simulink subsystem "EP_EmpennageForceMoment"  (R2025a)
settings: Solver=VariableStepAuto  StartTime=0.0  StopTime=10.0  RelTol=1e-3
undefined symbols (not defined in the file): EP_AirDensity_P, EP_CoGPos_P, EP_FinArea_P, EP_FinHeight_P, EP_FinLiftCoeffLim_P, EP_FinLiftSlope_P, EP_FinPos_P, EP_FinSetAng_P, EP_OutOfWakeAzimuth_P, EP_RotorRadius_P, EP_SkewAngleLwrLim_P, EP_SkewAngleUpprLim_P, EP_TailPlaneArea_P, EP_TailPlaneAzimuth_P, EP_TailPlaneLiftCoeffLim_P, EP_TailPlaneLiftSlope_P, EP_TailPlanePos_P, EP_TailPlaneSetAng_P, EP_WakeInitialInfluence_P
settings Model: DataDictionary=Empennage.sldd  EnableAccessToBaseWorkspace=off  DefaultTestHarness=EP_EmpennageForceMoment_Harness1  Creator=Admin  LastModifiedBy=Admin

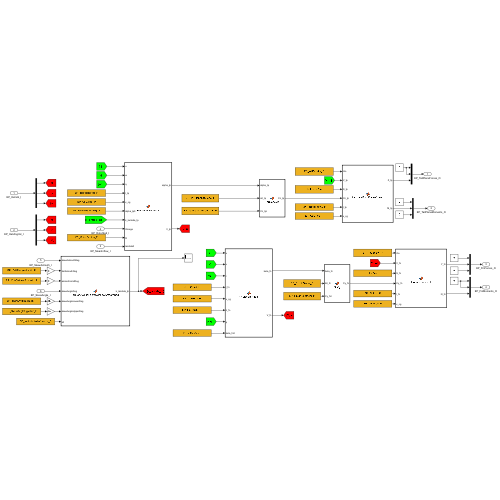
[thumbnail: Simulink's stored preview of the top-level diagram]
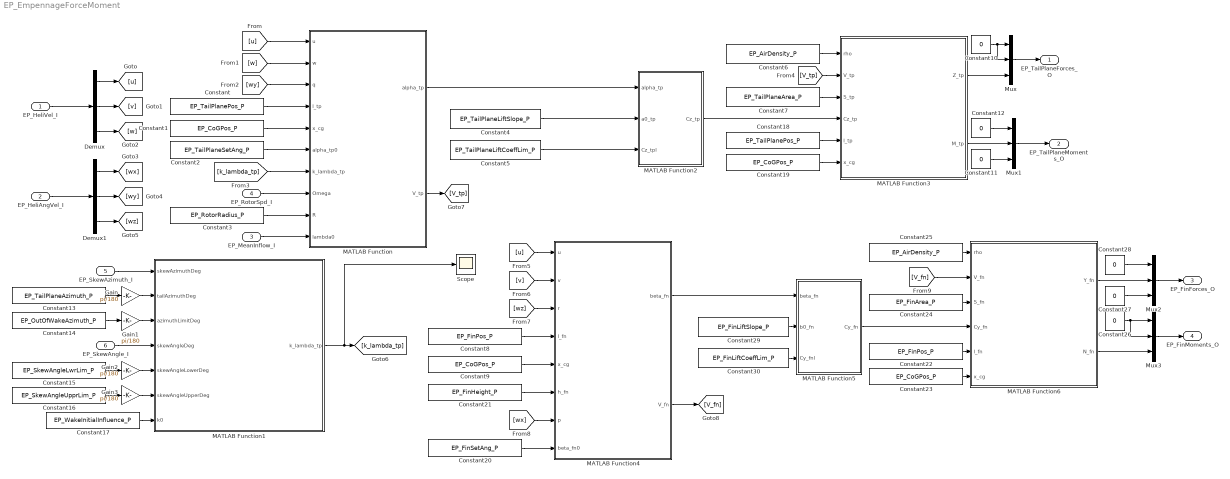
== system EP_EmpennageForceMoment ==
  EP_HeliVel_I : Inport
  EP_HeliAngVel_I : Inport  Port=2
  EP_MeanInflow_I : Inport  Port=3
  EP_RotorSpd_I : Inport  Port=4
  EP_SkewAzimuth_I : Inport  Port=5
  EP_SkewAngle_I : Inport  Port=6
  Constant : Constant  Value=EP_TailPlanePos_P
  Constant{1,9,19,23} (4 alike) : Constant  Value=EP_CoGPos_P  VectorParams1D=off
  Constant{10..12,26..28} (6 alike) : Constant  Value=0
  Constant13 : Constant  Value=EP_TailPlaneAzimuth_P
  Constant14 : Constant  Value=EP_OutOfWakeAzimuth_P
  Constant15 : Constant  Value=EP_SkewAngleLwrLim_P
  Constant16 : Constant  Value=EP_SkewAngleUpprLim_P
  Constant17 : Constant  Value=EP_WakeInitialInfluence_P
  Constant18 : Constant  Value=EP_TailPlanePos_P
  Constant2 : Constant  Value=EP_TailPlaneSetAng_P
  Constant20 : Constant  Value=EP_FinSetAng_P
  Constant21 : Constant  Value=EP_FinHeight_P
  Constant22 : Constant  Value=EP_FinPos_P
  Constant24 : Constant  Value=EP_FinArea_P
  Constant25 : Constant  Value=EP_AirDensity_P
  Constant29 : Constant  Value=EP_FinLiftSlope_P
  Constant3 : Constant  Value=EP_RotorRadius_P
  Constant30 : Constant  Value=EP_FinLiftCoeffLim_P
  Constant4 : Constant  Value=EP_TailPlaneLiftSlope_P
  Constant5 : Constant  Value=EP_TailPlaneLiftCoeffLim_P
  Constant6 : Constant  Value=EP_AirDensity_P
  Constant7 : Constant  Value=EP_TailPlaneArea_P
  Constant8 : Constant  Value=EP_FinPos_P
  Demux : Demux  Outputs=3
  Demux1 : Demux  Outputs=3
  Gain{,1..3} (4 alike) : Gain  Gain=pi/180
  MATLAB Function : MATLAB Function  TreatAsAtomicUnit=on
  MATLAB Function1 : MATLAB Function  TreatAsAtomicUnit=on
  MATLAB Function2 : MATLAB Function  TreatAsAtomicUnit=on
  MATLAB Function3 : MATLAB Function  TreatAsAtomicUnit=on
  MATLAB Function4 : MATLAB Function  TreatAsAtomicUnit=on
  MATLAB Function5 : MATLAB Function  TreatAsAtomicUnit=on
  MATLAB Function6 : MATLAB Function  TreatAsAtomicUnit=on
  Mux{,1..3} (4 alike) : Mux  Inputs=3
  Scope : Scope
      settings: ActiveDisplayYMinimum=-0.087499999999999981  ActiveDisplayYMaximum=0.7875  DataLoggingVariableName=ScopeData4
  EP_TailPlaneForces_O : Outport
  EP_TailPlaneMoments_O : Outport  Port=2
  EP_FinForces_O : Outport  Port=3
  EP_FinMoments_O : Outport  Port=4
  wires:
  EP_RotorSpd_I/1 -> MATLAB Function/8(Omega)
  EP_MeanInflow_I/1 -> MATLAB Function/10(lambda0)
  EP_SkewAngle_I/1 -> MATLAB Function1/4(skewAngleDeg)
  EP_SkewAzimuth_I/1 -> MATLAB Function1/1(skewAzimuthDeg)
  EP_HeliVel_I/1 -> Demux/1
  EP_HeliAngVel_I/1 -> Demux1/1
  Demux/1 -> [u]
  Demux/2 -> [v]
  Demux/3 -> [w]
  Demux1/1 -> [wx]
  Demux1/2 -> [wy]
  Demux1/3 -> [wz]
  [wy] -> MATLAB Function/3(q)
  [w] -> MATLAB Function/2(w)
  [u] -> MATLAB Function/1(u)
  Constant/1 -> MATLAB Function/4(l_tp)
  Constant1/1 -> MATLAB Function/5(x_cg)
  Constant2/1 -> MATLAB Function/6(alpha_tp0)
  MATLAB Function1/1(k_lambda_tp) -> [k_lambda_tp], Scope/1
  [k_lambda_tp] -> MATLAB Function/7(k_lambda_tp)
  Constant3/1 -> MATLAB Function/9(R)
  MATLAB Function/1(alpha_tp) -> MATLAB Function2/1(alpha_tp)
  MATLAB Function/2(V_tp) -> [V_tp]
  Constant4/1 -> MATLAB Function2/2(a0_tp)
  Constant5/1 -> MATLAB Function2/3(Cz_tpl)
  MATLAB Function2/1(Cz_tp) -> MATLAB Function3/4(Cz_tp)
  [V_tp] -> MATLAB Function3/2(V_tp)
  Constant6/1 -> MATLAB Function3/1(rho)
  Constant7/1 -> MATLAB Function3/3(S_tp)
  Constant18/1 -> MATLAB Function3/5(l_tp)
  Constant19/1 -> MATLAB Function3/6(x_cg)
  MATLAB Function3/1(Z_tp) -> Mux/3
  Constant10/1 -> Mux/2, Mux/1
  Mux/1 -> EP_TailPlaneForces_O/1
  Constant11/1 -> Mux1/3
  Constant12/1 -> Mux1/1
  Mux1/1 -> EP_TailPlaneMoments_O/1
  MATLAB Function3/2(M_tp) -> Mux1/2
  Constant13/1 -> Gain/1
  Constant14/1 -> Gain1/1
  Constant16/1 -> Gain3/1
  Constant17/1 -> MATLAB Function1/7(k0)
  Constant15/1 -> Gain2/1
  MATLAB Function4/1(beta_fn) -> MATLAB Function5/1(beta_fn)
  [u] -> MATLAB Function4/1(u)
  [v] -> MATLAB Function4/2(v)
  [wz] -> MATLAB Function4/3(r)
  Constant8/1 -> MATLAB Function4/4(l_fn)
  Constant20/1 -> MATLAB Function4/8(beta_fn0)
  Constant9/1 -> MATLAB Function4/5(x_cg)
  Constant21/1 -> MATLAB Function4/6(h_fn)
  [wx] -> MATLAB Function4/7(p)
  MATLAB Function5/1(Cy_fn) -> MATLAB Function6/4(Cy_fn)
  Constant22/1 -> MATLAB Function6/5(l_fn)
  Constant23/1 -> MATLAB Function6/6(x_cg)
  MATLAB Function4/2(V_fn) -> [V_fn]
  [V_fn] -> MATLAB Function6/2(V_fn)
  Constant25/1 -> MATLAB Function6/1(rho)
  Constant24/1 -> MATLAB Function6/3(S_fn)
  Constant26/1 -> Mux3/2, Mux3/1
  Mux3/1 -> EP_FinMoments_O/1
  MATLAB Function6/2(N_fn) -> Mux3/3
  Mux2/1 -> EP_FinForces_O/1
  MATLAB Function6/1(Y_fn) -> Mux2/2
  Constant28/1 -> Mux2/1
  Constant27/1 -> Mux2/3
  Constant29/1 -> MATLAB Function5/2(b0_fn)
  Constant30/1 -> MATLAB Function5/3(Cy_fnl)
  Gain/1 -> MATLAB Function1/2(tailAzimuthDeg)
  Gain1/1 -> MATLAB Function1/3(azimuthLimitDeg)
  Gain2/1 -> MATLAB Function1/5(skewAngleLowerDeg)
  Gain3/1 -> MATLAB Function1/6(skewAngleUpperDeg)

== matlab function EP_EmpennageForceMoment/MATLAB Function1 ==
  data: skewAzimuthDeg input; k_lambda_tp output; tailAzimuthDeg input; azimuthLimitDeg input; skewAngleDeg input; skewAngleLowerDeg input; skewAngleUpperDeg input; k0 input
function k_lambda_tp = TailplaneWakeFactorWindowSmoothDeg(skewAzimuthDeg, tailAzimuthDeg, ...
    azimuthLimitDeg, skewAngleDeg, skewAngleLowerDeg, skewAngleUpperDeg, k0)
% Smooth azimuth decay, hard skew-angle window

    dAzimuth = mod(skewAzimuthDeg - tailAzimuthDeg + 180, 360) - 180;

    if abs(dAzimuth) > azimuthLimitDeg
        azFactor = 0;
    else
        azFactor = 1 - abs(dAzimuth)/azimuthLimitDeg;
    end

    if skewAngleDeg > skewAngleLowerDeg && skewAngleDeg < skewAngleUpperDeg
        angleFactor = 1;
    else
        angleFactor = 0;
    end

    k_lambda_tp = k0 * azFactor * angleFactor;
end

== matlab function EP_EmpennageForceMoment/MATLAB Function ==
  data: u input; alpha_tp output; w input; q input; l_tp input; x_cg input; alpha_tp0 input; k_lambda_tp input; Omega input; R input; lambda0 input; V_tp output
function [alpha_tp, V_tp] = HorizontalStabAoA(u, w, q, l_tp, x_cg, alpha_tp0, k_lambda_tp, Omega, R, lambda0)
%HORIZONTALSTABAOA Compute horizontal stabilizer angle of attack.
%
% Equation:
%   alpha_tp = alpha_tp0 + atan( (w + q*(l_tp + x_cg) - k_lambda_tp*Omega*R*lambda0) / u ),   u >= 0
%
% Reverse-flow correction:
%   alpha_tp(reverse) = alpha_tp(forward) + pi,   u < 0
%
% Inputs:
%   u           - longitudinal body velocity at CG [m/s]
%   w           - vertical body velocity at CG [m/s]
%   q           - pitch rate [rad/s]
%   l_tp        - longitudinal distance from CG reference to tailplane arm [m]
%   x_cg        - CG offset used in model [m]
%   alpha_tp0   - tailplane setting / incidence angle [rad]
%   k_lambda_tp - tailplane rotor-wake interference coefficient [-]
%   Omega       - main rotor angular speed [rad/s]
%   R           - main rotor radius [m]
%   lambda0     - mean inflow ratio [-]
%
% Output:
%   alpha_tp    - horizontal stabilizer angle of attack [rad]
%
% Notes:
%   - Uses atan2 for better numerical robustness.
%   - For u < 0, applies the reverse-flow correction exactly as shown.
%   - Works with scalar or array inputs of compatible size.

    num = w + q .* (l_tp + x_cg) - k_lambda_tp .* Omega .* R .* lambda0;
    V_tp = sqrt(u^2 + num^2);
    % Forward-flow expression
    alpha_forward = alpha_tp0 + atan2(num, u);

    % Reverse-flow correction
    if u >= 0
        alpha_tp = alpha_forward;
    else
        alpha_tp = alpha_forward + pi;
    end
end

== matlab function EP_EmpennageForceMoment/MATLAB Function2 ==
  data: alpha_tp input; Cz_tp output; a0_tp input; Cz_tpl input
function Cz_tp = TailplaneCz(alpha_tp, a0_tp, Cz_tpl)
%TAILPLANECZ Calculate horizontal stabilizer Cz as in the paper.
%
% Inputs:
%   alpha_tp - tailplane angle of attack [rad]
%   a0_tp    - linear lift slope parameter
%   Cz_tpl   - saturation limit magnitude for Cz
%
% Output:
%   Cz_tp    - tailplane normal-force coefficient

    Cz_lin = -a0_tp .* sin(alpha_tp);

    if abs(Cz_lin) <= Cz_tpl
        Cz_tp = Cz_lin;
    else
        Cz_tp = -Cz_tpl * sign(sin(alpha_tp));
    end
end

== matlab function EP_EmpennageForceMoment/MATLAB Function3 ==
  data: rho input; Z_tp output; V_tp input; S_tp input; Cz_tp input; l_tp input; x_cg input; M_tp output
function [Z_tp, M_tp] = HorizontalStabForceMoment(rho, V_tp, S_tp, Cz_tp, l_tp, x_cg)
%#codegen
%HORIZONTALSTABFORCEMOMENT Calculate horizontal stabilizer force and moment.
%
% Equations:
%   Z_tp = 0.5 * rho * V_tp^2 * S_tp * Cz_tp
%   M_tp = (l_tp + x_cg) * Z_tp
%
% Inputs:
%   rho   - air density [kg/m^3]
%   V_tp  - tailplane effective airspeed [m/s]
%   S_tp  - horizontal stabilizer area [m^2]
%   Cz_tp - horizontal stabilizer force coefficient [-]
%   l_tp  - stabilizer arm from reference point [m]
%   x_cg  - CG offset [m]
%
% Outputs:
%   Z_tp  - stabilizer vertical force [N]
%   M_tp  - pitching moment about CG [N.m]

    Z_tp = 0.5 * rho * V_tp^2 * S_tp * Cz_tp;
    M_tp = (l_tp + x_cg) * Z_tp;
end

== matlab function EP_EmpennageForceMoment/MATLAB Function4 ==
  data: u input; beta_fn output; v input; r input; l_fn input; x_cg input; h_fn input; p input; beta_fn0 input; V_fn output
function [beta_fn, V_fn] = FinSideslipAngle(u, v, r, l_fn, x_cg, h_fn, p, beta_fn0)
%#codegen

v_eff_speed = v - r * (l_fn + x_cg);
v_eff_beta  = v - r * (l_fn + x_cg) + h_fn * p;

V_fn = sqrt(v_eff_speed^2 + u^2);

denom = V_fn;

if abs(denom) < 1e-9
    beta_fn = beta_fn0;
else
    arg = v_eff_beta / denom;

    if arg > 1
        arg = 1;
    elseif arg < -1
        arg = -1;
    end

    beta_fn = beta_fn0 + asin(arg);
end

== matlab function EP_EmpennageForceMoment/MATLAB Function5 ==
  data: beta_fn input; Cy_fn output; b0_fn input; Cy_fnl input
function Cy_fn = FinCy(beta_fn, b0_fn, Cy_fnl)
%#codegen
%FINCY Calculate vertical fin side-force coefficient Cy_fn.
%
% Equation:
%   Cy_lin = -b0_fn * sin(beta_fn)
%
% Saturation:
%   if |Cy_lin| <= Cy_fnl
%       Cy_fn = Cy_lin
%   else
%       Cy_fn = -Cy_fnl * sign(sin(beta_fn))
%   end
%
% Inputs:
%   beta_fn - fin effective sideslip angle [rad]
%   b0_fn   - linear side-force slope parameter [-]
%   Cy_fnl  - saturation limit magnitude of Cy_fn [-]
%
% Output:
%   Cy_fn   - fin side-force coefficient [-]

    Cy_lin = -b0_fn .* sin(beta_fn);

    if abs(Cy_lin) <= Cy_fnl
        Cy_fn = Cy_lin;
    else
        Cy_fn = -Cy_fnl * sign(sin(beta_fn));
    end
end

== matlab function EP_EmpennageForceMoment/MATLAB Function6 ==
  data: rho input; Y_fn output; V_fn input; S_fn input; Cy_fn input; l_fn input; x_cg input; N_fn output
function [Y_fn, N_fn] = FinForceMoment(rho, V_fn, S_fn, Cy_fn, l_fn, x_cg)
%#codegen
%FINFORCEMOMENT Calculate vertical fin side force and yawing moment.
%
% Equations:
%   Y_fn = 0.5 * rho * V_fn^2 * S_fn * Cy_fn
%   N_fn = -(l_fn + x_cg) * Y_fn
%
% Inputs:
%   rho   - air density [kg/m^3]
%   V_fn  - effective fin airspeed [m/s]
%   S_fn  - vertical fin area [m^2]
%   Cy_fn - fin side-force coefficient [-]
%   l_fn  - fin longitudinal arm [m]
%   x_cg  - CG offset [m]
%
% Outputs:
%   Y_fn  - fin side force [N]
%   N_fn  - fin yawing moment about CG [N*m]

    Y_fn = 0.5 * rho * V_fn^2 * S_fn * Cy_fn;
    N_fn = -(l_fn + x_cg) * Y_fn;
end
